simulink model "elements"  (R2014a)
settings: Solver=ode45  StartTime=0.0  StopTime=1  MaxStep=1e-5  RelTol=1e-5
libraries: powerlib x4
settings Model: Creator=mamta  LastModifiedBy=mamta

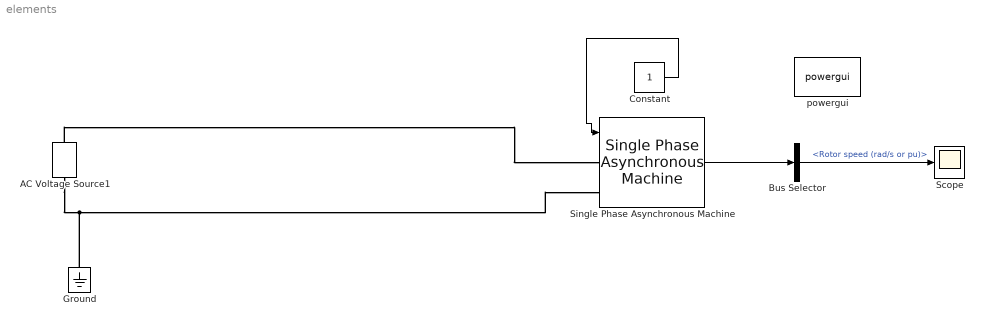
== system elements ==
  AC Voltage Source1 : powerlib/Electrical Sources/AC Voltage Source  Amplitude=220  Phase=0  Frequency=50  SampleTime=0  Measurements=None
  Bus Selector : BusSelector  OutputSignals=Mechanical.Rotor speed (rad/s or pu)
  Constant : Constant
  Ground : powerlib/Elements/Ground  LConnTagsString=a
  Scope : Scope
      settings: YMin=-2.75  YMax=-1.65  MaxDataPoints=1500000
  Single Phase Asynchronous Machine : powerlib/Machines/Single Phase Asynchronous Machine  MechanicalLoad=Torque Tm  UNITS=SI  MachineType=Split Phase  MeasurementBus=off  MainWindingStator="[2.02  7.4e-3]"  NominalParameters="[ .25*746  110  60]"  MainWindingRotor="[4.12  5.6e-3]"  MutualInductance=0.1772  AuxiliaryWinding="[7.14  8.5e-3]"  Mechanical="[0.0146  0  2 1.18]"  CapacitorStart="[2  254.7e-6]"  CapacitorRun="[18  21.1e-6]"  DisconnectionSpeed=75  InitialSpeed=0  DataType=SI  TsPowergui=0  TsBlock=-1
  powergui : powerlib/powergui  Priority=1  SimulationMode=Continuous  SolverType=Tustin  SampleTime=50e-6  frequency=60  SPID=off  DisableSnubberDevices=off  DisableRonSwitches=off  DisableVfSwitches=off  SwTol=0  Interpol=off  DisplayEquations=off  Ts=0  methode=off  frequencyindice=50  Pbase=100e6  ErrMax=1e-4  Iterations=50  UnitsV=kV  UnitsW=MW  FunctionMessages=off  echomessages=off  HookPort=off  EnableUseOfTLC=off  x0status=blocks  RestoreLinks=warning  ResistiveCurrentMeasurement=off  Frange=[0:2:500]  Ylog=off  Xlog=on  ShowGrid=off  save=off  variable=ZData  structure=0  ZoomFFT=off  StartTime=0.0  cycles=1  DisplayStyle=1  fundamental=60  FreqAxis=off  MaxFrequency=1000  frequencyindicesteady=1  RmsSteady=1  display=off
  wires:
  Single Phase Asynchronous Machine/1 -> Bus Selector/1
  Bus Selector/1 -> Scope/1  "<Rotor speed (rad/s or pu)>"
  Constant/1 -> Single Phase Asynchronous Machine/1
  connections:
  AC Voltage Source1/LConn1 -- Ground/LConn1 -- Single Phase Asynchronous Machine/LConn2
  AC Voltage Source1/RConn1 -- Single Phase Asynchronous Machine/LConn1
